simulink model "P_controller"  (R2021b)
settings: Solver=VariableStepAuto  StartTime=0.0  StopTime=20.0  RelTol=1e-3
settings Model: Creator=mahima  LastModifiedBy=mahima

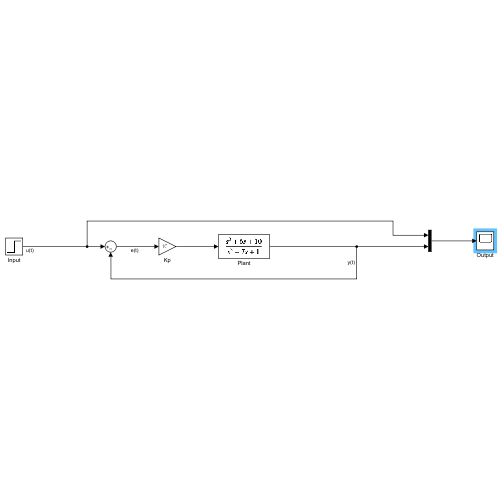
[thumbnail: Simulink's stored preview of the top-level diagram]
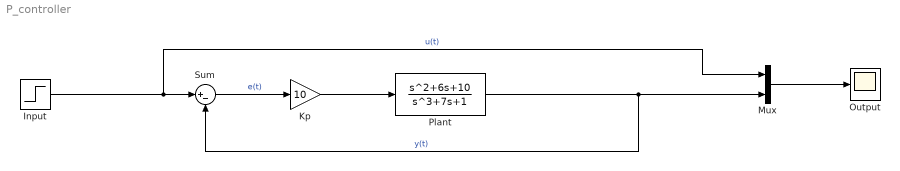
== system P_controller ==
  Input : Step  SampleTime=0
  Kp : Gain  Gain=10
  Mux : Mux  Inputs=2
  Output : Scope
  Plant : TransferFcn  Numerator=[1,6,10]  Denominator=[1,0,7,1]
  Sum : Sum  Inputs=|+-
  wires:
  Sum/1 -> Kp/1  "e(t)"
  Plant/1 -> Sum/2, Mux/2  "y(t)"
  Input/1 -> Mux/1, Sum/1  "u(t)"
  Mux/1 -> Output/1
  Kp/1 -> Plant/1
